simulink model "simulation"  (R2016a)
settings: Solver=VariableStepAuto  StartTime=0.0  StopTime=10.0  RelTol=1e-3
settings Model: Creator=AVAJANG-PC  LastModifiedBy=AVAJANG-PC

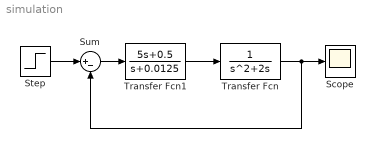
== system simulation ==
  Scope : Scope
  Step : Step  SampleTime=0
  Sum : Sum  Inputs=|+-
  Transfer Fcn : TransferFcn  Denominator=[1 2 0]
  Transfer Fcn1 : TransferFcn  Numerator=[5 0.5]  Denominator=[1 0.0125]
  wires:
  Transfer Fcn1/1 -> Transfer Fcn/1
  Sum/1 -> Transfer Fcn1/1
  Step/1 -> Sum/1
  Transfer Fcn/1 -> Sum/2, Scope/1
